simulink model "HybridPowertrain_TestBench_Final"  (R2017a)
settings: Solver=ode1  StartTime=0.0  StopTime=1400  FixedStep=0.01  RelTol=1e-3  EnableMultiTasking=on
undefined symbols (not defined in the file): AccActPos, air, Atm_temp, bms_inletair_temp, BMS_IstStrom, bms_maxchargecurrent, bms_maxdischargecurrent, BMS_Notfallkuehlung, BMS_SOC, BrkPdlPos, cal, Cells, Chg, D1_Commanded_Torque, D1_DC_Bus_Voltage, D2_Motor_Speed, D2_Torque_Feedback, DriverControls, EcoCAR3_Lib, Em, EngActStdyStTorq, Engine, EngSpd, env, ESS, fd, g, gb, Gearbox, GearBox, gps_lat, gps_long, Grade, I_loss, IMG, InstFuelConsmpRate, KeyPosition, lib_ESS_plant_V1_2, Loss, max_vehicle_rad_air_flow, mot, mph2kph, mph2ms, NeutralGear, ParkGear, PPEI_Engine_General_Status_2__ThrPos, PTEI_Engine_Torque_Status__EngActStdyStTorq, R_0, R_1, Ratio, RegenBrkDisable, rho, SampleTime, ShiftLeverPosition, SOC_bp, SOC_init, Spd, Speed, SW_CS_ON, SW_Engine_ON ... (+15)
libraries: simulink x39, fl_lib x13, nesl_utility x8, Utility x1, EC2_libraries x1
(part 4 of 5)

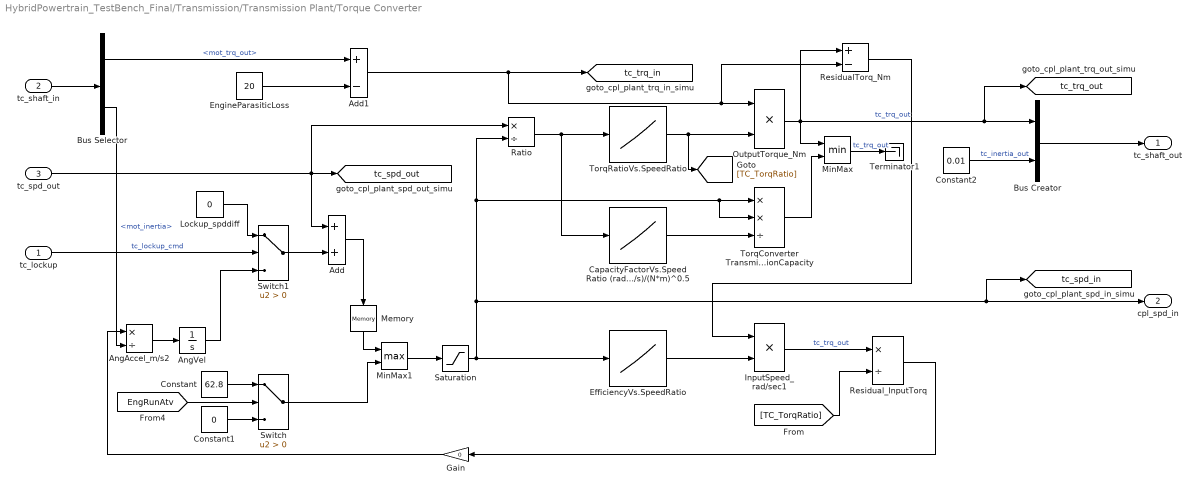
== system HybridPowertrain_TestBench_Final/Transmission/Transmission Plant/Torque Converter ==
  tc_lockup : Inport
  tc_shaft_in : Inport  Port=2
  tc_spd_out : Inport  Port=3
  Add : Sum
  Add1 : Sum  Inputs=+-
  AngAccel_m/s2 : Product  Inputs=*/
  AngVel : Integrator
  Bus Creator : BusCreator  Inputs=2
  Bus Selector : BusSelector  OutputSignals=mot_trq_out,mot_inertia
  CapacityFactorVs.SpeedRatio (rad/s)/(N*m)^0.5 : Lookup_n-D  NumberOfTableDimensions=1  BreakpointsForDimension1=[0 0.50 0.60 0.70 0.80 0.87 0.92 0.94 0.96 0.97]  Table=[12.2938 12.8588 13.1452 13.6285 14.6163 16.2675 19.3503 22.1046 29.9986 50.00]  InternalRulePriority=Speed  RndMeth=Simplest  InputSameDT=on
  Constant : Constant  Value=62.8
  Constant1 : Constant  Value=0
  Constant2 : Constant  Value=0.01
  EfficiencyVs.SpeedRatio : Lookup_n-D  NumberOfTableDimensions=1  BreakpointsForDimension1=[0 0.25 0.50 0.60 0.70 0.80 0.87 0.92 0.94 0.96 0.97 1.0]  Table="[0.10 0.50 0.70 0.8 0.8 0.80  0.85 0.87 0.91 0.95 0.96 0.96]"  InternalRulePriority=Speed  RndMeth=Simplest  InputSameDT=on
  EngineParasiticLoss : Constant  Value=20
  Gain : Gain  Gain=0
  InputSpeed_rad/sec1 : Product  Inputs=**
  Lockup_spddiff : Constant  Value=0
  Memory : Memory  X0=1
  MinMax : MinMax  Inputs=2
  MinMax1 : MinMax  Function=max  Inputs=2
  OutputTorque_Nm : Product  Inputs=**
  Ratio : Product  Inputs=*/
  ResidualTorq_Nm : Sum  Inputs=+-
  Residual_InputTorq : Product  Inputs=*/
  Saturation : Saturate  UpperLimit=1100  LowerLimit=1
  Switch : Switch  Criteria=u2 > Threshold
  Switch1 : Switch  Criteria=u2 > Threshold
  Terminator1 : Terminator
  TorqConverter TransmissionCapacity : Product  Inputs=**/
  TorqRatioVs.SpeedRatio : Lookup_n-D  NumberOfTableDimensions=1  BreakpointsForDimension1=[0 0.50 0.60 0.70 0.80 0.87 0.92 0.94 0.96 0.97]  Table=[2.2320 1.5462 1.4058 1.2746 1.1528 1.0732 1.0192 0.9983 0.9983 0.9983]  InternalRulePriority=Speed  RndMeth=Simplest  InputSameDT=on
  tc_shaft_out : Outport
  cpl_spd_in : Outport  Port=2
  tag scope: tc_spd_in=global, tc_spd_out=global, tc_trq_in=global, tc_trq_out=global
  wires:
  Add1/1 -> [tc_trq_in], ResidualTorq_Nm/2, OutputTorque_Nm/1
  Constant2/1 -> Bus Creator/2  "tc_inertia_out"
  tc_shaft_in/1 -> Bus Selector/1
  Bus Creator/1 -> tc_shaft_out/1
  Bus Selector/2 -> AngAccel_m/s2/2  "<mot_inertia>"
  tc_lockup/1 -> Switch1/2  "tc_lockup_cmd"
  TorqRatioVs.SpeedRatio/1 -> OutputTorque_Nm/2, [TC_TorqRatio]
  CapacityFactorVs.SpeedRatio (rad/s)/(N*m)^0.5/1 -> TorqConverter TransmissionCapacity/3
  Ratio/1 -> CapacityFactorVs.SpeedRatio (rad/s)/(N*m)^0.5/1, TorqRatioVs.SpeedRatio/1
  Saturation/1 -> Ratio/2, TorqConverter TransmissionCapacity/2, TorqConverter TransmissionCapacity/1, [tc_spd_in], cpl_spd_in/1, EfficiencyVs.SpeedRatio/1
  EfficiencyVs.SpeedRatio/1 -> InputSpeed_rad/sec1/2
  TorqConverter TransmissionCapacity/1 -> MinMax/2
  [TC_TorqRatio] -> Residual_InputTorq/2
  ResidualTorq_Nm/1 -> InputSpeed_rad/sec1/1
  InputSpeed_rad/sec1/1 -> Residual_InputTorq/1  "tc_trq_out"
  AngAccel_m/s2/1 -> AngVel/1
  AngVel/1 -> Switch1/3
  Memory/1 -> MinMax1/1
  EngineParasiticLoss/1 -> Add1/2
  Residual_InputTorq/1 -> Gain/1
  OutputTorque_Nm/1 -> ResidualTorq_Nm/1, Bus Creator/1, [tc_trq_out], MinMax/1  "tc_trq_out"
  MinMax/1 -> Terminator1/1  "tc_trq_out"
  tc_spd_out/1 -> Ratio/1, [tc_spd_out], Add/1
  Add/1 -> Memory/1
  Gain/1 -> AngAccel_m/s2/1
  MinMax1/1 -> Saturation/1
  Switch/1 -> MinMax1/2
  [EngRunAtv] -> Switch/2
  Constant/1 -> Switch/1
  Constant1/1 -> Switch/3
  Bus Selector/1 -> Add1/1  "<mot_trq_out>"
  Switch1/1 -> Add/2
  Lockup_spddiff/1 -> Switch1/1

== system HybridPowertrain_TestBench_Final/Wheels/Force calculation/Blending ==
  note: State dependent blending
  input : Inport
  Control (state) : Inport  Port=2
  Fcn : Fcn  Expr=(u<xl)*yl + (xl<=u)*(u<xc)*((yc-yl)*(u-xl)/(xc-xl)+yl) + (xc<=u)*(u<xr)*((yc-yr)*(u-xr)/(xc-xr)+yr) + (xr<=u)*yr
  Product : Product  SaturateOnIntegerOverflow=on  InputSameDT=on  OutDataTypeStr=Inherit: Same as first input
  Out1 : Outport
  wires:
  input/1 -> Product/1
  Control (state)/1 -> Fcn/1
  Product/1 -> Out1/1
  Fcn/1 -> Product/2

== system HybridPowertrain_TestBench_Final/Wheels/Force calculation/Rolling Resistance ==
  whl_spd : Inport
  grade : Inport  Port=2
  (N)^beta : Math  Operator=pow  SaturateOnIntegerOverflow=on
  (P)^alpha : Math  Operator=pow  SaturateOnIntegerOverflow=on
  Add2 : Sum  Inputs=+++
  Alpha_coeff : Constant  Value=Tire.Alpha
  Beta_coeff : Constant  Value=Tire.Beta
  Normal_Force : Gain  Gain=Vehicle.TestingMass*9.81
  Tire Pressure_N/m2 : Constant  Value=193053
  Tire Rolling Resistance : Product  Inputs=***
  Tire.A_coeff : Constant  Value=Tire.A_coeff
  Tire.B_coeff : Constant  Value=Tire.B_coeff
  Tire.C_coeff : Constant  Value=Tire.C_coeff
  Trigonometric Function : Trigonometry  Operator=cos
  Vtire*Coeff_B : Product  Inputs=**
  Vtire^2*Coeff_C : Product  Inputs=***
  rolling resistance : Outport
  wires:
  whl_spd/1 -> Vtire*Coeff_B/2, Vtire^2*Coeff_C/3, Vtire^2*Coeff_C/2
  grade/1 -> Trigonometric Function/1
  Tire Pressure_N/m2/1 -> (P)^alpha/1
  Alpha_coeff/1 -> (P)^alpha/2
  (P)^alpha/1 -> Tire Rolling Resistance/1
  Normal_Force/1 -> (N)^beta/1
  Beta_coeff/1 -> (N)^beta/2
  (N)^beta/1 -> Tire Rolling Resistance/2
  Tire.A_coeff/1 -> Add2/1
  Tire.B_coeff/1 -> Vtire*Coeff_B/1
  Tire.C_coeff/1 -> Vtire^2*Coeff_C/1
  Vtire^2*Coeff_C/1 -> Add2/3
  Vtire*Coeff_B/1 -> Add2/2
  Add2/1 -> Tire Rolling Resistance/3
  Tire Rolling Resistance/1 -> rolling resistance/1
  Trigonometric Function/1 -> Normal_Force/1

== system HybridPowertrain_TestBench_Final/ESS/ESS/Bosch_Li_Cell/Subsystem ==
  In1 : Inport
  In2 : Inport  Port=2
  Gain3 : Gain  Gain=I_loss
  Memory : Memory  InheritSampleTime=on
  Relational Operator : RelationalOperator  Operator=>  OutDataTypeStr=boolean  RndMeth=Nearest
  Switch : Switch
  Out1 : Outport
  wires:
  Gain3/1 -> Relational Operator/2, Switch/3
  In2/1 -> Gain3/1
  In1/1 -> Memory/1
  Relational Operator/1 -> Switch/2
  Switch/1 -> Out1/1
  Memory/1 -> Relational Operator/1, Switch/1

== system HybridPowertrain_TestBench_Final/ESS/ESS/Cooling_Loop1/Sensor ==
  Ideal Temperature Sensor : fl_lib/Thermal/Thermal Sensors/Ideal Temperature Sensor
      settings: SourceProductName=Simscape  SourceProductBaseCode=SS
  PS-Simulink Converter : nesl_utility/PS-Simulink Converter  PhysicalDomain=network_engine_domain  SubClassName=ps_output  LeftPortType=input  RightPortType=output  PseudoPeriodic=off  Frequencies=[]  Unit=1  AffineConversion=off
  Scope : Scope
  Thermal Reference : fl_lib/Thermal/Thermal Elements/Thermal Reference
  B : PMIOPort  Port=1  Side=Left
  wires:
  PS-Simulink Converter/1 -> Scope/1
  connections:
  B/RConn1 -- Ideal Temperature Sensor/LConn1
  Ideal Temperature Sensor/RConn1 -- Thermal Reference/LConn1
  PS-Simulink Converter/LConn1 -- Ideal Temperature Sensor/RConn2

== system HybridPowertrain_TestBench_Final/ESS/Soft BMS/BMS_HYB_1/BMS_HYB_02_BZ ==
  Constant : Constant
  Rolling Alive Counter : Stateflow chart  TreatAsAtomicUnit=on
  Switch : Switch  Criteria=u2 > Threshold
  Out1 : Outport
  wires:
  [BMS_CAN_fault] -> Switch/2
  Constant/1 -> Switch/1
  Rolling Alive Counter/1(RollingAliveCnt) -> Switch/3
  Switch/1 -> Out1/1  "BMS_HYB_02_BZ"

== system HybridPowertrain_TestBench_Final/ESS/Soft BMS/Energy Consumption/Divide by zero ==
  In1 : Inport
  Compare To Constant : simulink/Logic and Bit Operations/Compare To Constant  relop=<=  const=3.0  OutDataTypeStr=boolean
  Constant1 : Constant  Value=eps
  Switch2 : Switch  Criteria=u2 > Threshold
  Out1 : Outport
  wires:
  Constant1/1 -> Switch2/1
  Compare To Constant/1 -> Switch2/2
  In1/1 -> Switch2/3, Compare To Constant/1
  Switch2/1 -> Out1/1

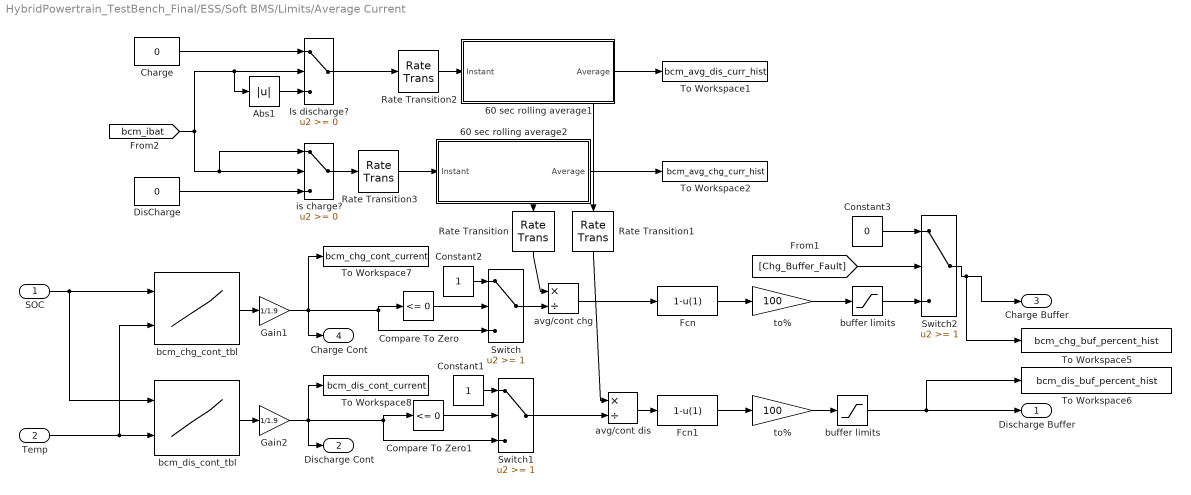
== system HybridPowertrain_TestBench_Final/ESS/Soft BMS/Limits/Average Current ==
  SOC : Inport
  Temp : Inport  Port=2
  60 sec rolling average1 : Subsystem
  60 sec rolling average2 : Subsystem
  Abs1 : Abs
  Charge : Constant  Value=0
  Compare To Zero : simulink/Logic and Bit Operations/Compare To Zero  relop=<=  OutDataTypeStr=boolean
  Compare To Zero1 : simulink/Logic and Bit Operations/Compare To Zero  relop=<=  OutDataTypeStr=boolean
  Constant1 : Constant
  Constant2 : Constant
  Constant3 : Constant  Value=0
  DisCharge : Constant  Value=0
  Fcn : Fcn  Expr=1-u(1)
  Fcn1 : Fcn  Expr=1-u(1)
  Gain1 : Gain  Gain=1/1.9
  Gain2 : Gain  Gain=1/1.9
  Is discharge? : Switch
  Rate Transition{,1..3} (4 alike) : RateTransition
  Switch : Switch  Threshold=1
  Switch1 : Switch  Threshold=1
  Switch2 : Switch  Threshold=1
  To Workspace1 : ToWorkspace  VariableName=bcm_avg_dis_curr_hist  SampleTime=-1
      settings: Decimation=WORKSPACE_DECIMATION
  To Workspace2 : ToWorkspace  VariableName=bcm_avg_chg_curr_hist  SampleTime=-1
      settings: Decimation=WORKSPACE_DECIMATION
  To Workspace5 : ToWorkspace  VariableName=bcm_chg_buf_percent_hist  SampleTime=-1
      settings: Decimation=WORKSPACE_DECIMATION
  To Workspace6 : ToWorkspace  VariableName=bcm_dis_buf_percent_hist  SampleTime=-1
      settings: Decimation=WORKSPACE_DECIMATION
  To Workspace7 : ToWorkspace  VariableName=bcm_chg_cont_current  SampleTime=-1
      settings: Decimation=WORKSPACE_DECIMATION
  To Workspace8 : ToWorkspace  VariableName=bcm_dis_cont_current  SampleTime=-1
      settings: Decimation=WORKSPACE_DECIMATION
  avg/cont chg : Product  Inputs=*/  RndMeth=Zero
  avg/cont dis : Product  Inputs=*/  RndMeth=Zero
  bcm_chg_cont_tbl : Lookup2D  RowIndex=ess.plant.init.limit.idx1_soc  ColumnIndex=ess.plant.init.limit.idx2_temp  Table=ess.plant.init.max_cont_charge
  bcm_dis_cont_tbl : Lookup2D  RowIndex=ess.plant.init.limit.idx1_soc  ColumnIndex=ess.plant.init.limit.idx2_temp  Table=ess.plant.init.max_cont_discharge
  buffer limits : Saturate  UpperLimit=100  LowerLimit=0
  "buffer limits " : Saturate  UpperLimit=100  LowerLimit=0
  is charge? : Switch
  to% : Gain  Gain=100
  "to% " : Gain  Gain=100
  Discharge Buffer : Outport
  Discharge Cont : Outport  Port=2
  Charge Buffer : Outport  Port=3
  Charge Cont : Outport  Port=4
  wires:
  [Chg_Buffer_Fault] -> Switch2/2
  Constant3/1 -> Switch2/1
  Switch2/1 -> To Workspace5/1, Charge Buffer/1
  buffer limits/1 -> Switch2/3
  Temp/1 -> bcm_dis_cont_tbl/2, bcm_chg_cont_tbl/2
  to%/1 -> buffer limits/1
  "to% "/1 -> "buffer limits "/1
  Fcn1/1 -> "to% "/1
  Fcn/1 -> to%/1
  avg/cont dis/1 -> Fcn1/1
  avg/cont chg/1 -> Fcn/1
  60 sec rolling average2/1(Average) -> To Workspace2/1, Rate Transition/1
  60 sec rolling average1/1(Average) -> To Workspace1/1, Rate Transition1/1
  is charge?/1 -> Rate Transition3/1
  Is discharge?/1 -> Rate Transition2/1
  DisCharge/1 -> is charge?/3
  Abs1/1 -> Is discharge?/3
  Charge/1 -> Is discharge?/1
  [bcm_ibat] -> is charge?/1, is charge?/2, Abs1/1, Is discharge?/2
  SOC/1 -> bcm_chg_cont_tbl/1, bcm_dis_cont_tbl/1
  Compare To Zero/1 -> Switch/2
  Constant2/1 -> Switch/1
  Switch/1 -> avg/cont chg/2
  bcm_chg_cont_tbl/1 -> Gain1/1
  Compare To Zero1/1 -> Switch1/2
  Constant1/1 -> Switch1/1
  Switch1/1 -> avg/cont dis/2
  bcm_dis_cont_tbl/1 -> Gain2/1
  "buffer limits "/1 -> To Workspace6/1, Discharge Buffer/1
  Gain1/1 -> To Workspace7/1, Compare To Zero/1, Switch/3, Charge Cont/1
  Gain2/1 -> Discharge Cont/1, Compare To Zero1/1, Switch1/3, To Workspace8/1
  Rate Transition/1 -> avg/cont chg/1
  Rate Transition1/1 -> avg/cont dis/1
  Rate Transition2/1 -> 60 sec rolling average1/1(Instant)
  Rate Transition3/1 -> 60 sec rolling average2/1(Instant)

== system HybridPowertrain_TestBench_Final/ESS/Soft BMS/Limits/Derate ==
  Current Limit : Inport
  Buffer : Inport  Port=2
  Cont Current : Inport  Port=3
  100A/sec : Gain  Gain=100*tloop
  Compare To Zero2 : simulink/Logic and Bit Operations/Compare To Zero  relop=<=  OutDataTypeStr=boolean
  Gain : Gain  Gain=-1
  Memory1 : Memory
  MinMax : MinMax  Function=max  Inputs=2
  StepTm[sec] : Constant  Value=tloop
  Sum : Sum  Inputs=|++
  Sum1 : Sum  Inputs=|-+
  Switch1 : Switch  Threshold=1
  Derate : Outport
  wires:
  Sum/1 -> Memory1/1, 100A/sec/1
  Switch1/1 -> Sum/1
  StepTm[sec]/1 -> Switch1/1
  Memory1/1 -> Gain/1, Sum/2
  Gain/1 -> Switch1/3
  Buffer/1 -> Compare To Zero2/1
  Compare To Zero2/1 -> Switch1/2
  100A/sec/1 -> Sum1/1
  Sum1/1 -> MinMax/1
  Current Limit/1 -> Sum1/2
  MinMax/1 -> Derate/1
  Cont Current/1 -> MinMax/2

== system HybridPowertrain_TestBench_Final/ESS/Soft BMS/Limits/Derate2 ==
  Buffer : Inport
  Cont Current : Inport  Port=2
  Current Limit : Inport  Port=3
  100A/sec : Gain  Gain=100*tloop
  Compare To Zero2 : simulink/Logic and Bit Operations/Compare To Zero  relop=<=  OutDataTypeStr=boolean
  Gain : Gain  Gain=-1
  Memory1 : Memory
  MinMax : MinMax  Function=max  Inputs=2
  StepTm[sec] : Constant  Value=tloop
  Sum : Sum  Inputs=|++
  Sum1 : Sum  Inputs=|-+
  Switch1 : Switch  Threshold=1
  Derate : Outport
  wires:
  Cont Current/1 -> MinMax/2
  MinMax/1 -> Derate/1
  Current Limit/1 -> Sum1/2
  Sum1/1 -> MinMax/1
  100A/sec/1 -> Sum1/1
  Compare To Zero2/1 -> Switch1/2
  Buffer/1 -> Compare To Zero2/1
  Gain/1 -> Switch1/3
  Memory1/1 -> Sum/2, Gain/1
  StepTm[sec]/1 -> Switch1/1
  Switch1/1 -> Sum/1
  Sum/1 -> 100A/sec/1, Memory1/1

== system HybridPowertrain_TestBench_Final/ICE Simple/Engine Plant Modified/Core Engine/Core Engine ==
  note: Engine.DisplacedVolume
  Engine Speed (RPM) : Inport
  CO : Lookup2D  RowIndex=Engine.Engine.Emissions.SPEED  ColumnIndex=Engine.Engine.Emissions.TQ  Table=Engine.Engine.Emissions.CO/1000  LookUpMeth=Interpolation-Use End Values
  CO2 : Lookup2D  RowIndex=Engine.Engine.Emissions.SPEED  ColumnIndex=Engine.Engine.Emissions.TQ  Table=Engine.Engine.Emissions.CO2/1000  LookUpMeth=Interpolation-Use End Values
  Fuel Flow : Lookup2D  RowIndex=Engine.Engine.FuelFlow.SPEED  ColumnIndex=Engine.Engine.FuelFlow.TQ  Table=Engine.Engine.FuelFlow.FuelFlow  LookUpMeth=Interpolation-Use End Values
  HC : Lookup2D  RowIndex=Engine.Engine.Emissions.SPEED  ColumnIndex=Engine.Engine.Emissions.TQ  Table=Engine.Engine.Emissions.HC/1000  LookUpMeth=Interpolation-Use End Values
  Half of Displacement : Gain  Gain=2.4/(2*1000)
  Ideal Gas Constant R : Gain  Gain=0.287
  Kg/s to g/s : Gain  Gain=1000
  Manifold_Dynamics_Model : Subsystem
  Memory : Memory
  NOx : Lookup2D  RowIndex=Engine.Engine.Emissions.SPEED  ColumnIndex=Engine.Engine.Emissions.TQ  Table=Engine.Engine.Emissions.NOx/1000  LookUpMeth=Interpolation-Use End Values
  Power Enrichment Torque Boundary vs Speed : Lookup_n-D  NumberOfTableDimensions=1  BreakpointsForDimension1=Engine.Engine.PEBound.SPEED  Table=Engine.Engine.PEBound.PEBound  ExtrapMethod=Clip  InternalRulePriority=Speed  RndMeth=Simplest  InputSameDT=on
  Product : Product  Inputs=***
  RPM to RPS : Gain  Gain=1/60
  Relational Operator : RelationalOperator  Operator=>  OutDataTypeStr=boolean  RndMeth=Nearest
  Speed-Density Mass Flow : Product  Inputs=*/
  Tamb_K : Constant  Value=293.15
  Torque : Lookup2D  RowIndex=Engine.Engine.TQ.SPEED  ColumnIndex=Engine.Engine.TQ.MAF  Table=Engine.Engine.TQ.TQ  LookUpMeth=Interpolation-Use End Values
  Volumetric Efficiency : Lookup2D  RowIndex=Engine.Engine.VE.MAP  ColumnIndex=Engine.Engine.VE.SPEED  Table=Engine.Engine.VE.VE  LookUpMeth=Interpolation-Use End Values
  Brake Torque (Nm) : Outport
  Fuel Flow (g/s) : Outport  Port=2
  PE Status : Outport  Port=3
  HC (g/s) : Outport  Port=4
  CO (g/s) : Outport  Port=5
  NOx (g/s) : Outport  Port=6
  CO2 (g/s) : Outport  Port=7
  Intake Port Airflow (g/s) : Outport  Port=8
  wires:
  Torque/1 -> Brake Torque (Nm)/1, Relational Operator/1, Memory/1  "Brake Torque"
  [INTAKEPORTFLOW] -> Torque/2
  Fuel Flow/1 -> Fuel Flow (g/s)/1  "Fuel Flow"
  Memory/1 -> CO2/2, NOx/2, CO/2, HC/2, Fuel Flow/2
  Power Enrichment Torque Boundary vs Speed/1 -> Relational Operator/2
  Relational Operator/1 -> PE Status/1
  HC/1 -> HC (g/s)/1
  CO/1 -> CO (g/s)/1
  NOx/1 -> NOx (g/s)/1
  CO2/1 -> CO2 (g/s)/1
  [INTAKEPORTFLOW] -> Intake Port Airflow (g/s)/1
  Volumetric Efficiency/1 -> Product/1
  Ideal Gas Constant R/1 -> Speed-Density Mass Flow/2
  Product/1 -> Speed-Density Mass Flow/1
  Tamb_K/1 -> Ideal Gas Constant R/1
  RPM to RPS/1 -> Half of Displacement/1
  Half of Displacement/1 -> Product/2
  Engine Speed (RPM)/1 -> Torque/1, Fuel Flow/1, HC/1, CO/1, NOx/1, Power Enrichment Torque Boundary vs Speed/1, CO2/1, RPM to RPS/1, Volumetric Efficiency/2
  [ThrPosCmd_int] -> Manifold_Dynamics_Model/1(In1)
  Manifold_Dynamics_Model/1(MAP_kg/s) -> Product/3, Volumetric Efficiency/1  "MAP"
  Kg/s to g/s/1 -> [INTAKEPORTFLOW]
  Speed-Density Mass Flow/1 -> Kg/s to g/s/1, Manifold_Dynamics_Model/2(In2)

== system HybridPowertrain_TestBench_Final/ICE Simple/Engine Plant Modified/Core Engine/Crank Process/function ==
  EngSpd : Inport
  f : TriggerPort  TriggerType=function-call  VariantControl=Variant
      settings: CopyFcn=Stateflow.SLINSF.SimulinkMan.removeBlockPreDeleteFcn  PreDeleteFcn=Stateflow.SLINSF.SimulinkMan.unsafePredeleteFcn
  1-D Lookup Table : Lookup_n-D  NumberOfTableDimensions=1  BreakpointsForDimension1=[0 50 120 210 300 320 340 350 400]  Table=[90 90 90 90 90 90 90 90 90]  InternalRulePriority=Speed  RndMeth=Simplest  InputSameDT=on
  Sine Wave : Sin  Amplitude=20  Frequency=41.88
  Sum : Sum
  CrankTrq : Outport
  wires:
  1-D Lookup Table/1 -> Sum/1
  EngSpd/1 -> 1-D Lookup Table/1
  Sum/1 -> CrankTrq/1
  Sine Wave/1 -> Sum/2

== system HybridPowertrain_TestBench_Final/ICE Simple/Engine Plant Modified/Core Engine/EngEfficiency ==
  note: Mechanical Power [W]
  Torque : Inport
  Speed : Inport  Port=2
  Fuel Consumption : Inport  Port=3
  Divide by Zero Fix : Subsystem
  Divide_by_Zero_Fix1 : EC2_libraries/Divide_by_Zero_Fix  Commented=on
  From1 : From  Commented=on  GotoTag=Wh_out
  From2 : From  Commented=on  GotoTag=Wh_in
  Goto1 : Goto  Commented=on  GotoTag=Wh_out
  Goto2 : Goto  Commented=on  GotoTag=Wh_in
  Integrator1 : Integrator  Commented=on  LimitOutput=on  LowerSaturationLimit=0
  Integrator2 : Integrator  Commented=on  LimitOutput=on  LowerSaturationLimit=0
  OnlyPositiveEnergy : Saturate  Commented=on  UpperLimit=inf  LowerLimit=0
  Percentage Efficiency : Gain  Gain=100
  Product : Product  RndMeth=Zero
  "RPM to rad/s " : Gain  Gain=pi/30
  Scope : Scope  NumInputPorts=2
  Specific Energy LHV in J/kg : Gain  Gain=Engine.Fuel.Lower_Heating_Value/1000
  Sum : Sum  Inputs=-+
  To Workspace7 : ToWorkspace  Commented=on  VariableName=eng_Wh_pos_eff_hist  SampleTime=-1
      settings: Decimation=WORKSPACE_DECIMATION
  engine_efficiency : Scope
  limit_efficiency[0-100%] : Saturate  UpperLimit=100  LowerLimit=0
  PowerLoss : Outport
  wires:
  limit_efficiency[0-100%]/1 -> engine_efficiency/1
  Sum/1 -> PowerLoss/1  "Losses [W]"
  Fuel Consumption/1 -> Specific Energy LHV in J/kg/1
  Specific Energy LHV in J/kg/1 -> Divide by Zero Fix/2(Divide), Sum/2, Integrator2/1, Scope/2  "Thermal Power [W]"
  Torque/1 -> Product/2  "Nm"
  Speed/1 -> "RPM to rad/s "/1  "rpm"
  Percentage Efficiency/1 -> limit_efficiency[0-100%]/1  "Efficiency [%]"
  Divide by Zero Fix/1(Output) -> Percentage Efficiency/1
  Product/1 -> Scope/1, Divide by Zero Fix/1(Multiply), OnlyPositiveEnergy/1, Sum/1  "wer [W]"
  Divide_by_Zero_Fix1/1 -> To Workspace7/1
  From1/1 -> Divide_by_Zero_Fix1/1
  From2/1 -> Divide_by_Zero_Fix1/2
  Integrator1/1 -> Goto1/1
  OnlyPositiveEnergy/1 -> Integrator1/1
  Integrator2/1 -> Goto2/1
  "RPM to rad/s "/1 -> Product/1

== system HybridPowertrain_TestBench_Final/ICE Simple/Engine Plant Modified/Core Engine/EngineThermal ==
  note: Temp Delta C deg
  PowerLoss : Inport
  Divide : Product  Inputs=*/
  Divide1 : Product  Inputs=**
  Engine Mass : Constant  Value=Engine.Mass
  Memory : Memory  X0=Engine.Init_T_amb
  Memory1 : Memory
  Product : Product  RndMeth=Zero
  Specific Heat Cap Aluminum : Constant  Value=Engine.Specific_Heat
  Sum : Sum  Inputs=|++
  Sum1 : Sum  Inputs=|+-
  tloop : Constant  Value=0.01
  Temp[degC] : Outport
  tag scope: Heat_Transfer_Eng=global
  wires:
  Memory1/1 -> Sum1/2
  Divide1/1 -> Divide/1  "J"
  Sum1/1 -> Divide1/2
  Memory/1 -> Sum/2
  PowerLoss/1 -> Sum1/1, [Heat_Transfer_Eng]  "J/s"
  Engine Mass/1 -> Product/1  "kg"
  Specific Heat Cap Aluminum/1 -> Product/2  "J/kg*K"
  Product/1 -> Divide/2
  Sum/1 -> Memory/1, Temp[degC]/1
  Divide/1 -> Sum/1
  tloop/1 -> Divide1/1
  [Heat_Reject_Eng] -> Memory1/1

== system HybridPowertrain_TestBench_Final/ICE Simple/Engine Plant Modified/Radiator/Divide by Zero Fix ==
  Multiply : Inport
  Divide : Inport  Port=2
  Compare To Zero : simulink/Logic and Bit Operations/Compare To Zero  relop=<=  OutDataTypeStr=boolean
  Constant1 : Constant  Value=0
  Constant2 : Constant
  Product2 : Product  Inputs=/*  SaturateOnIntegerOverflow=on  InputSameDT=on  OutDataTypeStr=Inherit: Same as first input
  Switch : Switch  Threshold=1
  Switch1 : Switch  Threshold=1
  Output : Outport
  wires:
  Multiply/1 -> Product2/2
  Switch1/1 -> Output/1
  Constant1/1 -> Switch1/1
  Product2/1 -> Switch1/3
  Switch/1 -> Product2/1
  Divide/1 -> Switch/3, Compare To Zero/1
  Constant2/1 -> Switch/1
  Compare To Zero/1 -> Switch1/2, Switch/2

== system HybridPowertrain_TestBench_Final/ICE Simple/Soft ECM/Fuel Consumption/Divide by Zero Fix ==
  Divide : Inport
  Multiply : Inport  Port=2
  Compare To Zero : simulink/Logic and Bit Operations/Compare To Zero  relop=<=  OutDataTypeStr=boolean
  Constant1 : Constant  Value=0
  Constant2 : Constant
  Product2 : Product  Inputs=/*  SaturateOnIntegerOverflow=on  InputSameDT=on  OutDataTypeStr=Inherit: Same as first input
  Switch : Switch  Threshold=1
  Switch1 : Switch  Threshold=1
  Output : Outport
  wires:
  Multiply/1 -> Product2/2
  Switch1/1 -> Output/1
  Constant1/1 -> Switch1/1
  Product2/1 -> Switch1/3
  Switch/1 -> Product2/1
  Divide/1 -> Compare To Zero/1, Switch/3
  Constant2/1 -> Switch/1
  Compare To Zero/1 -> Switch1/2, Switch/2

== system HybridPowertrain_TestBench_Final/ICE Simple/Soft ECM/Fuel Consumption/Divide by Zero Fix1 ==
  Divide : Inport
  Multiply : Inport  Port=2
  Compare To Zero : simulink/Logic and Bit Operations/Compare To Zero  relop=<=  OutDataTypeStr=boolean
  Constant1 : Constant  Value=0
  Constant2 : Constant
  Product2 : Product  Inputs=/*  SaturateOnIntegerOverflow=on  InputSameDT=on  OutDataTypeStr=Inherit: Same as first input
  Switch : Switch  Threshold=1
  Switch1 : Switch  Threshold=1
  Output : Outport
  wires:
  Compare To Zero/1 -> Switch/2, Switch1/2
  Constant2/1 -> Switch/1
  Divide/1 -> Compare To Zero/1, Switch/3
  Switch/1 -> Product2/1
  Product2/1 -> Switch1/3
  Constant1/1 -> Switch1/1
  Switch1/1 -> Output/1
  Multiply/1 -> Product2/2

== system HybridPowertrain_TestBench_Final/IMG/IMG Plant/Calculate Mot Efficiency, MotPwrMech, and, MotPwrElec/Lower Limit ==
  In1 : Inport
  Constant3 : Constant  Value=Lolimit
  MinMax : MinMax  Function=max  Inputs=2
  Out1 : Outport
  wires:
  In1/1 -> MinMax/1
  Constant3/1 -> MinMax/2
  MinMax/1 -> Out1/1

== system HybridPowertrain_TestBench_Final/IMG/IMG Plant/Calculate Mot Efficiency, MotPwrMech, and, MotPwrElec/MCUOverTemp Fault ==
  In1 : Inport
  Gain : Gain  Gain=3
  Switch : Switch  Threshold=1
  Out1 : Outport
  wires:
  In1/1 -> Switch/3, Gain/1
  [MCUOverTemp] -> Switch/2
  Gain/1 -> Switch/1
  Switch/1 -> Out1/1

== system HybridPowertrain_TestBench_Final/IMG/IMG Plant/Motor_Plant/Efficiency Calcs ==
  Speed_rpm : Inport
  Torq_cmd_Nm : Inport  Port=2
  Batt_volt : Inport  Port=3
  Abs1 : Abs
  Constant : Constant
  Constant1 : Constant  Value=0
  Current_consum : Product  Inputs=*/
  Efficiency Map : Lookup_n-D  BreakpointsForDimension1=mot.map.trqindex  BreakpointsForDimension2=mot.map.spdindex  Table=mot.map.eff  InternalRulePriority=Speed  RndMeth=Simplest  InputSameDT=on
  Electrical power motoring : Product  Inputs=*//
  Electrical power regen : Product  Inputs=***
  Gain : Gain  Gain=2*3.14/60
  Gain1 : Gain  Gain=-1
  MCU_eff : Constant  Value=0.97
  Mech_power : Product  Inputs=**
  MinMax : MinMax  Function=max  Inputs=2
  MinMax1 : MinMax  Function=max  Inputs=2
  Saturation : Saturate  UpperLimit=400  LowerLimit=-400
  Switch : Switch  Criteria=u2 > Threshold
  Switch1 : Switch  Criteria=u2 > Threshold  Threshold=100
  min_eff : Constant  Value=0.1
  Mot_current : Outport
  Mech_power_W : Outport  Port=2
  Elec_power_W : Outport  Port=3
  wires:
  Speed_rpm/1 -> Efficiency Map/2, Gain/1
  Torq_cmd_Nm/1 -> Mech_power/2, Abs1/1, Switch/2
  Electrical power regen/1 -> Switch/3
  MinMax/1 -> Electrical power motoring/2, Electrical power regen/2
  Current_consum/1 -> Gain1/1
  Saturation/1 -> Mot_current/1  "Mot_current_A"
  Gain/1 -> Mech_power/1
  Batt_volt/1 -> Switch1/2, MinMax1/1
  Abs1/1 -> Efficiency Map/1
  Mech_power/1 -> Electrical power motoring/1, Electrical power regen/1, Mech_power_W/1  "Mech_power_W"
  MCU_eff/1 -> Electrical power regen/3, Electrical power motoring/3
  Electrical power motoring/1 -> Switch/1
  min_eff/1 -> MinMax/2
  Switch1/1 -> Elec_power_W/1, Current_consum/1  "Elec_power_W"
  Efficiency Map/1 -> MinMax/1
  MinMax1/1 -> Current_consum/2
  Constant/1 -> MinMax1/2
  Gain1/1 -> Saturation/1  "Mot_current_A"
  Switch/1 -> Switch1/1  "Elec_power_W"
  Constant1/1 -> Switch1/3

== system HybridPowertrain_TestBench_Final/IMG/IMG Plant/Thermal/Motor Thermal ==
  In1 : Inport
  Add1 : Sum  Inputs=+-
  Add2 : Sum
  Divide : Product  Inputs=*/
  Lower Limit : Subsystem  mask{Lolimit=t_amb+20}
      mask prompts: Lolimit "Lower Limit"
  Memory1 : Memory
  Motor Mass : Constant  Value=mot.plant.init.motor_mass
  Product : Product  RndMeth=Zero
  "Pump " : Constant  Value=0
  Specific Heat Cap Aluminum : Constant  Value=mot.plant.init.specific_heat
  tloop : Gain  Gain=tloop
  Out1 : Outport
  wires:
  Specific Heat Cap Aluminum/1 -> Product/2  "J/kg*K"
  Product/1 -> Divide/2
  Memory1/1 -> Add2/2
  Add2/1 -> Lower Limit/1(In1)
  Lower Limit/1(Out1) -> Out1/1, Memory1/1
  Divide/1 -> Add2/1
  tloop/1 -> Divide/1  "J"
  Motor Mass/1 -> Product/1  "kg"
  "Pump "/1 -> Add1/2
  In1/1 -> Add1/1
  Add1/1 -> tloop/1

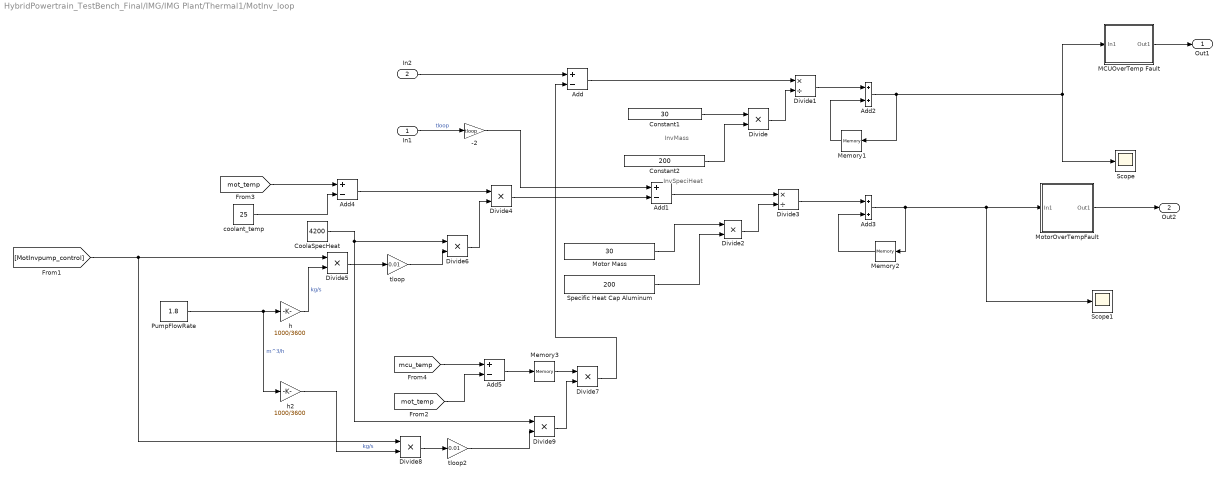
== system HybridPowertrain_TestBench_Final/IMG/IMG Plant/Thermal1/MotInv_loop ==
  note: InvSpeciHeat
  note: InvMass
  In1 : Inport
  In2 : Inport  Port=2
  -2 : Gain  Gain=tloop
  Add{,1,4..5} (4 alike) : Sum  Inputs=+-
  Add2 : Sum
  Add3 : Sum
  Constant1 : Constant  Value=30
  Constant2 : Constant  Value=200
  CoolaSpecHeat : Constant  Value=4200
  Divide{,2,4..9} (8 alike) : Product  Inputs=**
  Divide1 : Product  Inputs=*/
  Divide3 : Product  Inputs=*/
  MCUOverTemp Fault : Subsystem
  Memory1 : Memory  X0=25
  Memory2 : Memory  X0=25
  Memory3 : Memory
  Motor Mass : Constant  Value=30
  MotorOverTempFault : Subsystem
  PumpFlowRate : Constant  Value=1.8
  Scope : Scope
  Scope1 : Scope
  Specific Heat Cap Aluminum : Constant  Value=200
  coolant_temp : Constant  Value=25
  h : Gain  Gain=1000/3600
  h2 : Gain  Gain=1000/3600
  tloop : Gain  Gain=0.01
  tloop2 : Gain  Gain=0.01
  Out1 : Outport
  Out2 : Outport  Port=2
  wires:
  Add1/1 -> Divide3/1
  Memory1/1 -> Add2/2
  coolant_temp/1 -> Add4/2
  Divide/1 -> Divide1/2
  Specific Heat Cap Aluminum/1 -> Divide2/2
  Constant1/1 -> Divide/1
  Add/1 -> Divide1/1
  Memory2/1 -> Add3/2
  Add4/1 -> Divide4/1
  Add3/1 -> Scope1/1, MotorOverTempFault/1(In1), Memory2/1
  Divide6/1 -> Divide4/2
  Divide3/1 -> Add3/1
  Divide5/1 -> tloop/1
  Add2/1 -> MCUOverTemp Fault/1(In1), Scope/1, Memory1/1
  Divide2/1 -> Divide3/2
  Constant2/1 -> Divide/2
  Motor Mass/1 -> Divide2/1
  Divide1/1 -> Add2/1
  Divide7/1 -> Add/2
  h/1 -> Divide5/2  "kg/s"
  tloop/1 -> Divide6/2
  CoolaSpecHeat/1 -> Divide6/1, Divide9/1
  PumpFlowRate/1 -> h2/1, h/1  "m^3/h"
  h2/1 -> Divide8/2  "kg/s"
  Divide9/1 -> Divide7/2
  Divide8/1 -> tloop2/1
  tloop2/1 -> Divide9/2
  Divide4/1 -> Add1/2
  Add5/1 -> Memory3/1
  Memory3/1 -> Divide7/1
  MCUOverTemp Fault/1(Out1) -> Out1/1
  MotorOverTempFault/1(Out1) -> Out2/1
  [mot_temp] -> Add4/1
  [mcu_temp] -> Add5/1
  [mot_temp] -> Add5/2
  In1/1 -> -2/1  "tloop"
  In2/1 -> Add/1
  -2/1 -> Add1/1
  [MotInvpump_control] -> Divide8/1, Divide5/1

== system HybridPowertrain_TestBench_Final/IMG/IMG Plant/Thermal1/Motor Thermal ==
  In1 : Inport
  Add1 : Sum  Inputs=+-
  Add2 : Sum
  Divide : Product  Inputs=*/
  Lower Limit : Subsystem  mask{Lolimit=t_amb+20}
      mask prompts: Lolimit "Lower Limit"
  Memory1 : Memory
  Motor Mass : Constant  Value=mot.plant.init.motor_mass
  Product : Product  RndMeth=Zero
  "Pump " : Constant  Value=0
  Specific Heat Cap Aluminum : Constant  Value=mot.plant.init.specific_heat
  tloop : Gain  Gain=tloop
  Out1 : Outport
  wires:
  Specific Heat Cap Aluminum/1 -> Product/2  "J/kg*K"
  Product/1 -> Divide/2
  Memory1/1 -> Add2/2
  Add2/1 -> Lower Limit/1(In1)
  Lower Limit/1(Out1) -> Out1/1, Memory1/1
  Divide/1 -> Add2/1
  tloop/1 -> Divide/1  "J"
  Motor Mass/1 -> Product/1  "kg"
  "Pump "/1 -> Add1/2
  In1/1 -> Add1/1
  Add1/1 -> tloop/1

== system HybridPowertrain_TestBench_Final/IMG/IMG Plant/Torque Calculation/electric machine filter ==
  trq : Inport
  Interval Test : simulink/Logic and Bit Operations/Interval Test  IntervalClosedRight=on  uplimit=0.5  IntervalClosedLeft=on  lowlimit=-0.5  OutDataTypeStr=boolean
  Switch : Switch  Threshold=0.5
  electric machine time response : TransferFcn  Denominator=[mot.plant.init.time_response 1]
  filtered : Outport
  wires:
  electric machine time response/1 -> Switch/3
  Interval Test/1 -> Switch/2
  trq/1 -> Interval Test/1, electric machine time response/1, Switch/1
  Switch/1 -> filtered/1

== system HybridPowertrain_TestBench_Final/IMG/IMG Plant/Torque Calculation/max torque  ==
  cmd : Inport
  speed : Inport  Port=2
  Memory : Memory
  Peak trq max - Motoring : Lookup  InputValues=mot.plant.init.regen.trq_max.idx1_spd  Table=mot.plant.init.motor.trq_max.map  LookUpMeth=Interpolation-Use End Values  SaturateOnIntegerOverflow=on
  Peak trq max - Regen : Lookup  InputValues=mot.plant.init.regen.trq_max.idx1_spd  Table=mot.plant.init.regen.trq_max.map  LookUpMeth=Interpolation-Use End Values  SaturateOnIntegerOverflow=on
  Switch1 : Switch  SaturateOnIntegerOverflow=on
  rad/s  to RPM : Gain  Gain=30/pi
  max torque : Outport
  wires:
  Peak trq max - Motoring/1 -> Switch1/1
  speed/1 -> rad/s  to RPM/1
  cmd/1 -> Switch1/2
  Switch1/1 -> max torque/1
  Memory/1 -> Peak trq max - Motoring/1, Peak trq max - Regen/1
  rad/s  to RPM/1 -> Memory/1
  Peak trq max - Regen/1 -> Switch1/3

== system HybridPowertrain_TestBench_Final/IMG/Soft MCU/Torque Calculation/max torque  ==
  Req : Inport
  speed : Inport  Port=2
  torque : Inport  Port=3
  2-D Lookup Table : Lookup_n-D  Commented=on  BreakpointsForDimension1=mot.plant.init.eff_trq.idx2_trq  BreakpointsForDimension2=mot.plant.init.eff_trq.idx1_spd  Table=mot.plant.init.eff_trq.map  InternalRulePriority=Speed  RndMeth=Simplest  InputSameDT=on
  Abs : Abs  SaturateOnIntegerOverflow=on
  Abs1 : Abs  Commented=on
  Abs2 : Abs  Commented=on
  Constant : Constant  Commented=on  Value=84500
  Cont trq max - Motoring : Lookup  InputValues=mot.plant.init.motor.trq_cont.idx1_spd  Table=mot.plant.init.motor.trq_cont.map  LookUpMeth=Interpolation-Use End Values  SaturateOnIntegerOverflow=on
  Cont trq max - Regen : Lookup  InputValues=mot.plant.init.regen.trq_cont.idx1_spd  Table=mot.plant.init.regen.trq_cont.map  LookUpMeth=Interpolation-Use End Values  SaturateOnIntegerOverflow=on
  Divide : Product  Commented=on  Inputs=**/
  Divide by zero : Subsystem  Commented=on
  Gain2 : Gain  Commented=on  Gain=1/100
  Heat index : Subsystem
  Memory : Memory
  Peak trq max - Motoring : Lookup  Commented=on  InputValues=mot.plant.init.regen.trq_max.idx1_spd  Table=mot.plant.init.motor.trq_max.map  LookUpMeth=Interpolation-Use End Values  SaturateOnIntegerOverflow=on
  Peak trq max - Motoring1 : Lookup  InputValues=mot.plant.init.regen.trq_max.idx1_spd  Table=mot.plant.init.motor.trq_max.map  LookUpMeth=Interpolation-Use End Values  SaturateOnIntegerOverflow=on
  Peak trq max - Regen : Lookup  InputValues=mot.plant.init.regen.trq_max.idx1_spd  Table=mot.plant.init.regen.trq_max.map  LookUpMeth=Interpolation-Use End Values  SaturateOnIntegerOverflow=on
  Product2 : Product  SaturateOnIntegerOverflow=on  InputSameDT=on  OutDataTypeStr=Inherit: Same as first input
  Product3 : Product  SaturateOnIntegerOverflow=on  InputSameDT=on  OutDataTypeStr=Inherit: Same as first input
  Product5 : Product  SaturateOnIntegerOverflow=on  InputSameDT=on  OutDataTypeStr=Inherit: Same as first input
  RPM to rad/s : Gain  Commented=on  Gain=pi/30
  Sign : Signum
  Sum : Sum  SaturateOnIntegerOverflow=on  InputSameDT=on  OutDataTypeStr=Inherit: Same as first input
  Sum1 : Sum  Inputs=-+  SaturateOnIntegerOverflow=on  InputSameDT=on  OutDataTypeStr=Inherit: Same as first input
  Switch : Switch  SaturateOnIntegerOverflow=on
  Switch1 : Switch  SaturateOnIntegerOverflow=on
  cst : Constant
  max torque : Outport
  wires:
  Heat index/1(Heat index) -> Product2/2, Sum1/1
  cst/1 -> Sum1/2
  Product3/1 -> Sum/2
  Sum1/1 -> Product3/1
  Product2/1 -> Sum/1
  Switch1/1 -> Product3/2
  Switch/1 -> Heat index/1(cont torque), Product2/1
  Peak trq max - Regen/1 -> Switch1/3
  Cont trq max - Regen/1 -> Switch/3
  Cont trq max - Motoring/1 -> Switch/1
  torque/1 -> Heat index/2(torque)
  Abs/1 -> Product5/2
  Sum/1 -> Abs/1, Sign/1
  Product5/1 -> max torque/1
  Sign/1 -> Product5/1
  Memory/1 -> Cont trq max - Motoring/1, Cont trq max - Regen/1, Peak trq max - Motoring1/1, Peak trq max - Regen/1
  speed/1 -> Memory/1
  Constant/1 -> Divide/1
  RPM to rad/s/1 -> Divide by zero/1(In1)
  Abs2/1 -> 2-D Lookup Table/2
  Abs1/1 -> 2-D Lookup Table/1
  2-D Lookup Table/1 -> Gain2/1
  Gain2/1 -> Divide/2
  Req/1 -> Switch/2, Switch1/2
  Divide by zero/1(Out1) -> Divide/3
  Peak trq max - Motoring1/1 -> Switch1/1

== system HybridPowertrain_TestBench_Final/Transmission/Soft TCM/6L45 Logic/Gearbox_Control.Shift_Schedule.PlotShiftSchedule/Subsystem ==

== system HybridPowertrain_TestBench_Final/Transmission/Transmission Plant/Gearbox/Inertia Calculation ==
  Inertia_in : Inport
  gear number : Inport  Port=2
  Product2 : Product  Inputs=3  SaturateOnIntegerOverflow=on  InputSameDT=on  OutDataTypeStr=Inherit: Same as first input
  Sum : Sum  Inputs=|++  SaturateOnIntegerOverflow=on  InputSameDT=on  OutDataTypeStr=Inherit: Same as first input
  Sum2 : Sum  Inputs=|++  SaturateOnIntegerOverflow=on  InputSameDT=on  OutDataTypeStr=Inherit: Same as first input
  Switch : Switch  Criteria=u2 ~= 0  Threshold=0.5  SaturateOnIntegerOverflow=on  InputSameDT=on
  gb_inertia_in : Constant  Value=Gearbox.InputShaftInertia
  gb_inertia_out : Constant  Value=Gearbox.OutputShaftInertia
  gear ratio table : Lookup  InputValues=gb.plant.init.ratio.idx1_gear  Table=gb.plant.init.ratio.map  OutDataTypeStr=double  SaturateOnIntegerOverflow=on
  Inertia : Outport
  wires:
  gear ratio table/1 -> Product2/1, Product2/2
  Sum2/1 -> Switch/1
  Inertia_in/1 -> Sum/1
  Product2/1 -> Sum2/1
  gb_inertia_in/1 -> Sum/2
  Sum/1 -> Product2/3
  gb_inertia_out/1 -> Sum2/2, Switch/3
  gear number/1 -> Switch/2, gear ratio table/1
  Switch/1 -> Inertia/1

== system HybridPowertrain_TestBench_Final/Transmission/Transmission Plant/Gearbox/Speed Calculation ==
  note: +(u[1]==1)*u[2]
  gear number : Inport
  spd out : Inport  Port=2
  torque input : Inport  Port=3
  Inertia Input : Inport  Port=4
  Fcn2 : Fcn  Expr=(u[1]==0)*u[4]+(u[1]>0)*u[3]
  Mux : Mux
  P/N : Subsystem
  Product : Product  SaturateOnIntegerOverflow=on  InputSameDT=on  OutDataTypeStr=Inherit: Same as first input
  R/D : Subsystem
  gear ratio table : Lookup  InputValues=gb.plant.init.ratio.idx1_gear  Table=gb.plant.init.ratio.map  SaturateOnIntegerOverflow=on
  Speed : Outport
  wires:
  Mux/1 -> Fcn2/1
  gear number/1 -> Mux/1, P/N/3(gear), R/D/2(gear number), gear ratio table/1
  torque input/1 -> P/N/1(torque input)
  Inertia Input/1 -> P/N/2(Inertia Input)
  spd out/1 -> Product/1
  gear ratio table/1 -> Product/2
  Product/1 -> Mux/2, R/D/1(spd in), P/N/4(inital speed)
  P/N/1(speed) -> Mux/4, R/D/3(speed1)
  R/D/1(spd in filtered) -> Mux/3, Speed/1

== system HybridPowertrain_TestBench_Final/Transmission/Transmission Plant/Gearbox/Subsystem ==
  In1 : Inport
  In2 : Inport  Port=2
  Add : Sum
  Constant : Constant  Value=200
  Switch2 : Switch  Criteria=u2 > Threshold
  Out1 : Outport
  wires:
  Add/1 -> Switch2/1
  Constant/1 -> Add/1
  [Brk_Flt] -> Switch2/2
  In2/1 -> Switch2/3
  In1/1 -> Add/2
  Switch2/1 -> Out1/1

== system HybridPowertrain_TestBench_Final/Transmission/Transmission Plant/Gearbox/Subsystem1 ==
  speed out : Inport
  gear number : Inport  Port=2
  " input torque" : Inport  Port=3
  1-D Lookup Table : Lookup_n-D  NumberOfTableDimensions=1  BreakpointsForDimension1=[0 1 8000]  Table=[0 5.5 15]  InternalRulePriority=Speed  RndMeth=Simplest  InputSameDT=on
  Abs : Abs  SaturateOnIntegerOverflow=on
  Abs1 : Abs  SaturateOnIntegerOverflow=on
  Abs2 : Abs  SaturateOnIntegerOverflow=on
  Blending (state dependent) : Subsystem  mask(State dependent blending){xl=-gb.plant.init.spd_thr, yl=-1, xc=0, yc=0, xr=gb.plant.init.spd_thr, yr=1}
      mask prompts: xl "Left point (x):"; yl "Left point (y):"; xc "Center point (x):"; yc "Center point (y):"; xr "Right point (x):"; yr "Right point (y):"
      mask help: This block implements state dependent smoothing/blending. IMPORTANT: See help menu.
      mask Help: The output equals the product of the first input and a "hat" function defined by the three points specified in the dialog box.  The second input forms the argument to the hat function.\n\nIMPORTANT: A divide by zero error will result if first coordinates of the three points specified for the hat function are NOT distinct.
      mask Display: plot([-1 1 3 6 8], [1.5 1.5 0.5 4.0 4.0])
  Gain : Gain  Gain=10
  Product5 : Product  SaturateOnIntegerOverflow=on  InputSameDT=on  OutDataTypeStr=Inherit: Same as first input
  Product6 : Product  SaturateOnIntegerOverflow=on  InputSameDT=on  OutDataTypeStr=Inherit: Same as first input
  Saturation1 : Saturate  UpperLimit=inf  LowerLimit=min( gb.plant.init.trq_loss.idx1_trq )
  Saturation2 : Saturate  UpperLimit=inf  LowerLimit=min( gb.plant.init.trq_loss.idx2_spd )
  Saturation3 : Saturate  UpperLimit=8  LowerLimit=1
  Sum1 : Sum  Inputs=+-  SaturateOnIntegerOverflow=on  InputSameDT=on  OutDataTypeStr=Inherit: Same as first input
  Torque loss : Lookup_n-D  NumberOfTableDimensions=3  BreakpointsForDimension1=gb.plant.init.trq_loss.idx1_trq  BreakpointsForDimension2=gb.plant.init.trq_loss.idx2_spd  BreakpointsForDimension3=gb.plant.init.trq_loss.idx3_gear  Table=gb.plant.init.trq_loss.map
  gear ratio table : Lookup  InputValues=gb.plant.init.ratio.idx1_gear  Table=gb.plant.init.ratio.map  SaturateOnIntegerOverflow=on
  torque_out : Outport
  wires:
  Saturation2/1 -> Torque loss/2
  Saturation1/1 -> Torque loss/1
  Abs/1 -> Saturation1/1
  Product5/1 -> Blending (state dependent)/2(Control (state)), Abs1/1  "dtr_trans_speed"
  Abs1/1 -> Saturation2/1
  speed out/1 -> 1-D Lookup Table/1, Product5/1
  Product6/1 -> torque_out/1
  Blending (state dependent)/1(Output) -> Gain/1
  Sum1/1 -> Product6/2
  " input torque"/1 -> Sum1/1, Abs/1
  gear number/1 -> Abs2/1, gear ratio table/1
  Gain/1 -> Sum1/2
  gear ratio table/1 -> Product5/2, Product6/1
  Abs2/1 -> Saturation3/1
  Saturation3/1 -> Torque loss/3
  1-D Lookup Table/1 -> Blending (state dependent)/1(Input)

== system HybridPowertrain_TestBench_Final/Transmission/Transmission Plant/Gearbox/Torque calculation ==
  speed out : Inport
  gear number : Inport  Port=2
  " input torque" : Inport  Port=3
  Abs : Abs  Commented=on  SaturateOnIntegerOverflow=on
  Abs1 : Abs  Commented=on  SaturateOnIntegerOverflow=on
  Abs2 : Abs  Commented=on  SaturateOnIntegerOverflow=on
  Abs3 : Abs
  Blending (state dependent) : Subsystem  mask(State dependent blending){xl=-gb.plant.init.spd_thr, yl=-1, xc=0, yc=0, xr=gb.plant.init.spd_thr, yr=1}
      mask prompts: xl "Left point (x):"; yl "Left point (y):"; xc "Center point (x):"; yc "Center point (y):"; xr "Right point (x):"; yr "Right point (y):"
      mask help: This block implements state dependent smoothing/blending. IMPORTANT: See help menu.
      mask Help: The output equals the product of the first input and a "hat" function defined by the three points specified in the dialog box.  The second input forms the argument to the hat function.\n\nIMPORTANT: A divide by zero error will result if first coordinates of the three points specified for the hat function are NOT distinct.
      mask Display: plot([-1 1 3 6 8], [1.5 1.5 0.5 4.0 4.0])
  Constant : Constant  Value=2
  Constant1 : Constant
  Constant2 : Constant  Value=5.5
  Efficiency : Gain  Gain=0.85
  Gain : Gain
  ParasiticLoss : Lookup_n-D  Commented=on  BreakpointsForDimension1=Ratio  BreakpointsForDimension2=Spd  Table=Loss  InternalRulePriority=Speed  RndMeth=Simplest  InputSameDT=on
  Product1 : Product  Inputs=**/  SaturateOnIntegerOverflow=on  InputSameDT=on  OutDataTypeStr=Inherit: Same as first input
  Product5 : Product  SaturateOnIntegerOverflow=on  InputSameDT=on  OutDataTypeStr=Inherit: Same as first input
  Product6 : Product  SaturateOnIntegerOverflow=on  InputSameDT=on  OutDataTypeStr=Inherit: Same as first input
  Saturation1 : Saturate  Commented=on  UpperLimit=inf  LowerLimit=min( gb.plant.init.trq_loss.idx1_trq )
  Saturation2 : Saturate  Commented=on  UpperLimit=inf  LowerLimit=min( gb.plant.init.trq_loss.idx2_spd )
  Saturation3 : Saturate  Commented=on  UpperLimit=8  LowerLimit=1
  Scope : Scope
  Sum1 : Sum  Inputs=+-  SaturateOnIntegerOverflow=on  InputSameDT=on  OutDataTypeStr=Inherit: Same as first input
  Switch : Switch  Criteria=u2 > Threshold
  Torque loss : Lookup_n-D  Commented=on  NumberOfTableDimensions=3  BreakpointsForDimension1=gb.plant.init.trq_loss.idx1_trq  BreakpointsForDimension2=gb.plant.init.trq_loss.idx2_spd  BreakpointsForDimension3=gb.plant.init.trq_loss.idx3_gear  Table=gb.plant.init.trq_loss.map
  gear ratio table : Lookup  InputValues=gb.plant.init.ratio.idx1_gear  Table=gb.plant.init.ratio.map  SaturateOnIntegerOverflow=on
  torque_out : Outport
  wires:
  Saturation2/1 -> Torque loss/2
  Saturation1/1 -> Torque loss/1
  Abs/1 -> Saturation1/1
  Product5/1 -> ParasiticLoss/2, Blending (state dependent)/2(Control (state)), Abs1/1  "dtr_trans_speed"
  Abs1/1 -> Saturation2/1
  speed out/1 -> Product5/1
  Product6/1 -> Efficiency/1
  Blending (state dependent)/1(Output) -> Gain/1
  Sum1/1 -> Product6/2
  " input torque"/1 -> Sum1/1, Abs/1
  gear number/1 -> Abs3/1, Abs2/1, gear ratio table/1
  gear ratio table/1 -> Switch/1, Switch/2, Product5/2, Product6/1
  Abs2/1 -> Saturation3/1
  Saturation3/1 -> Torque loss/3
  Constant2/1 -> Blending (state dependent)/1(Input)
  Abs3/1 -> ParasiticLoss/1
  Efficiency/1 -> Scope/1, torque_out/1
  Gain/1 -> Product1/1
  Constant/1 -> Product1/2
  Product1/1 -> Sum1/2
  Switch/1 -> Product1/3
  Constant1/1 -> Switch/3

== system HybridPowertrain_TestBench_Final/ESS/Soft BMS/Limits/Average Current/60 sec rolling average1 ==
  Instant : Inport
  1 second : Delay  DelayLength=1/tloop  InputProcessing=Inherited  SampleTime=tloop
  1sec trigger : Subsystem
  60 sec average : Subsystem
  Gain1 : Gain  Gain=tloop
  Rate Transition : RateTransition
  Sum1 : Sum  Inputs=++-
  accumulate : Memory  InheritSampleTime=on
  accumulate1 : Memory  InheritSampleTime=on
  Average : Outport
  wires:
  accumulate1/1 -> Average/1
  60 sec average/1(Average) -> accumulate1/1
  accumulate/1 -> Sum1/1
  1 second/1 -> Sum1/3
  Instant/1 -> Sum1/2, 1 second/1
  Sum1/1 -> Gain1/1, accumulate/1
  1sec trigger/1(Trigger) -> 60 sec average/Enable
  Gain1/1 -> Rate Transition/1
  Rate Transition/1 -> 60 sec average/1(1sec)

== system HybridPowertrain_TestBench_Final/ESS/Soft BMS/Limits/Average Current/60 sec rolling average2 ==
  Instant : Inport
  1 second : Delay  DelayLength=1/tloop  InputProcessing=Inherited  SampleTime=tloop
  1sec trigger : Subsystem
  60 sec average : Subsystem
  Gain1 : Gain  Gain=tloop
  Rate Transition : RateTransition
  Sum1 : Sum  Inputs=++-
  accumulate : Memory  InheritSampleTime=on
  accumulate1 : Memory  InheritSampleTime=on
  Average : Outport
  wires:
  Sum1/1 -> accumulate/1, Gain1/1
  Instant/1 -> 1 second/1, Sum1/2
  1 second/1 -> Sum1/3
  accumulate/1 -> Sum1/1
  60 sec average/1(Average) -> accumulate1/1
  accumulate1/1 -> Average/1
  1sec trigger/1(Trigger) -> 60 sec average/Enable
  Gain1/1 -> Rate Transition/1
  Rate Transition/1 -> 60 sec average/1(1sec)

== system HybridPowertrain_TestBench_Final/ICE Simple/Engine Plant Modified/Core Engine/Core Engine/Manifold_Dynamics_Model ==
  note: Throttle_air flow
  In1 : Inport
  In2 : Inport  Port=2
  (2/(k+1))^(k/(k-1)) : Fcn  Expr=(2/(u(1)+1))^(u(1)/(u(1)-1))
  Bus Creator : BusCreator  Inputs=2
  Bus Creator1 : BusCreator  Inputs=2
  CA vs TP : Lookup  InputValues=Engine.Throttle.CA.TPP  Table=Engine.Throttle.CA.CA  LookUpMeth=Interpolation-Use End Values
  Cd : Constant  Value=0.82
  ETC Actuator Dynamics : TransferFcn  Denominator=[0.1 1]
  Fcn1 : Fcn  Expr=(u(2)^(2/u(1)))-(u(2)^((u(1)+1)/u(1)))
  Fcn2 : Fcn  Expr=(((u(1)-1)/(2*u(1)))*(2/(u(1)+1))^((u(1)+1)/(u(1)-1)))
  Fcn3 : Fcn  Expr=((u(1))*(u(2)))^0.5
  Fcn4 : Fcn  Expr=sqrt(2*u(1)/(u(1)-1))
  Gain : Gain  Gain=0.75
  Integrator : Integrator  InitialCondition=101325
  K : Constant  Value=1.4
  MAP' : Product  Inputs=***/
  Mat : Product  Inputs=*****/
  Memory : Memory
  Pamb : Constant  Value=101325
  Pr : Product  Inputs=*/
  R : Constant  Value=8.31447
  Relational Operator : RelationalOperator  OutDataTypeStr=boolean  RndMeth=Nearest
  Tamb_K : Constant  Value=293.15
  Vi_m3 : Constant  Value=0.001
  beta2 : Switch  Criteria=u2 > Threshold
  g/s to kg/s : Gain  Gain=1/1000
  mat-map : Sum  Inputs=+-
  MAP_kg/s : Outport
  wires:
  In1/1 -> ETC Actuator Dynamics/1
  Mat/1 -> mat-map/1  "mat"
  MAP'/1 -> Memory/1
  Vi_m3/1 -> MAP'/4
  [B] -> MAP'/2
  [A] -> MAP'/3
  Fcn4/1 -> Mat/5
  Tamb_K/1 -> Bus Creator1/2, [A]
  [C] -> Pr/1
  R/1 -> Bus Creator1/1, [B]
  CA vs TP/1 -> Gain/1
  Cd/1 -> Mat/2
  Relational Operator/1 -> beta2/2
  Bus Creator1/1 -> Fcn3/1
  Pamb/1 -> Pr/2, Mat/1
  Fcn3/1 -> Mat/6
  Fcn2/1 -> beta2/3
  (2/(k+1))^(k/(k-1))/1 -> Relational Operator/2
  beta2/1 -> Mat/4
  Bus Creator/1 -> Fcn1/1, Fcn2/1, Fcn4/1
  Pr/1 -> Bus Creator/2, Relational Operator/1
  K/1 -> Bus Creator/1, (2/(k+1))^(k/(k-1))/1
  Fcn1/1 -> beta2/1
  mat-map/1 -> MAP'/1
  In2/1 -> mat-map/2
  Memory/1 -> Integrator/1
  g/s to kg/s/1 -> MAP_kg/s/1
  ETC Actuator Dynamics/1 -> CA vs TP/1
  Integrator/1 -> [C], g/s to kg/s/1
  Gain/1 -> Mat/3

== system HybridPowertrain_TestBench_Final/ICE Simple/Engine Plant Modified/Core Engine/EngEfficiency/Divide by Zero Fix ==
  Multiply : Inport
  Divide : Inport  Port=2
  Compare To Zero : simulink/Logic and Bit Operations/Compare To Zero  relop=<=  OutDataTypeStr=boolean
  Constant1 : Constant  Value=0
  Constant2 : Constant
  Product2 : Product  Inputs=/*  SaturateOnIntegerOverflow=on  InputSameDT=on  OutDataTypeStr=Inherit: Same as first input
  Switch : Switch  Threshold=1
  Switch1 : Switch  Threshold=1
  Output : Outport
  wires:
  Multiply/1 -> Product2/2
  Switch1/1 -> Output/1
  Constant1/1 -> Switch1/1
  Product2/1 -> Switch1/3
  Switch/1 -> Product2/1
  Divide/1 -> Switch/3, Compare To Zero/1
  Constant2/1 -> Switch/1
  Compare To Zero/1 -> Switch1/2, Switch/2

== system HybridPowertrain_TestBench_Final/IMG/IMG Plant/Thermal/Motor Thermal/Lower Limit ==
  In1 : Inport
  Constant3 : Constant  Value=Lolimit
  MinMax : MinMax  Function=max  Inputs=2
  Out1 : Outport
  wires:
  In1/1 -> MinMax/1
  Constant3/1 -> MinMax/2
  MinMax/1 -> Out1/1

== system HybridPowertrain_TestBench_Final/IMG/IMG Plant/Thermal1/MotInv_loop/MCUOverTemp Fault ==
  In1 : Inport
  Gain : Gain  Gain=3
  Switch : Switch  Threshold=1
  Out1 : Outport
  wires:
  In1/1 -> Switch/3, Gain/1
  [MCUOverTemp] -> Switch/2
  Gain/1 -> Switch/1
  Switch/1 -> Out1/1

== system HybridPowertrain_TestBench_Final/IMG/IMG Plant/Thermal1/MotInv_loop/MotorOverTempFault ==
  In1 : Inport
  Gain : Gain  Gain=2
  Switch1 : Switch  Threshold=1
  Out1 : Outport
  wires:
  In1/1 -> Gain/1, Switch1/3
  [MotOverTemp] -> Switch1/2
  Gain/1 -> Switch1/1
  Switch1/1 -> Out1/1

== system HybridPowertrain_TestBench_Final/IMG/IMG Plant/Thermal1/Motor Thermal/Lower Limit ==
  In1 : Inport
  Constant3 : Constant  Value=Lolimit
  MinMax : MinMax  Function=max  Inputs=2
  Out1 : Outport
  wires:
  In1/1 -> MinMax/1
  Constant3/1 -> MinMax/2
  MinMax/1 -> Out1/1
